simulink model "controller_v13"  (R2020b)
settings: Solver=ode4  StartTime=0.0  StopTime=inf  RelTol=1e-3
undefined symbols (not defined in the file): ctr, DiscIntNeverNeededParam, flt, IO397, mdl, rbt, rsim, som, ukf_P0_flat, ukf_prediction_time, ukf_s0, ukf_sys, ukf_use_prediction
libraries: simulink x31, slrealtimeloglib x5, slrealtimeseriallib x5, speedgoatlib_fpga_analog_io x4, slrealtimetgmanagement x3, speedgoatlib_fpga x2, speedgoatlib_fpga_dio x1, slrealtimeutilitieslib x1
(part 4 of 5)

== matlab function controller_v13/Adaptive Controller/ICRA'23 attitude and thrust MPC controller -> It works/Geometric Attitude Controller ==
  data: time input; cmd_B_torque output; R input; Omega input; Rd input; Omegad input; tau_ext input; ctr parameter; rbt parameter; mdl parameter; att_e output
function [cmd_B_torque, att_e]   = fcn(time, R, Omega, Rd, Omegad, tau_ext, ctr, rbt, mdl)
%#codegen
% r: curr pos
% r_dot: curr vel
% R: current attitude
% Omega: current body rates
% rd : des pos
% rd_d: des vel
% Rd: desired attitude (rotation matrix)
% Omegad: desired angular velocity


% current attitude
R = get_rotation_matrix(R);     % transform vector in rotation matrix
Omega = Omega(:);
Omegad = Omegad(:);

% desired attitude & angvel
Rd = get_rotation_matrix(Rd);
% inertial frame 3-axis



% thrust magnitude control, eq 19
%A = -ctr.lee.pos.kx*ex - ctr.lee.pos.kv*ev - rbt.m*mdl.g*e3; % + P.mass*xd_2dot;
%cmd_B_acc_z = dot(-A, R*e3)/rbt.m;

Rd = get_desired_attitude_x_axis(Rd, R);
%Rd = get_desired_attitude_y_axis(Rd, R);

% inertia matrix
J = diag([ctr.lee.ixx, ctr.lee.iyy, ctr.lee.izz]);

% attitude and angular velocity errors
eR     = (1/2)*vee(Rd.'*R - R.'*Rd);
eOmega = Omega - R.'*Rd*Omegad;
% desired torque
M = -ctr.lee.kR*eR - ctr.lee.kOmega*eOmega + cross(Omega, J*Omega)...
    - J*(hat(Omega)*R.'*Rd*Omegad) ...
    - ctr.torque_obs.factor.*[tau_ext(1); tau_ext(2); 0.0]; % ...
  % - J*(- R.'*Rd*Omegad_1dot);
  % - J*(hat(Omega)*R.'*Rd*Omegad) ...

%att_e = eR'*eR; % squared norm of the error
att_e = eR;
cmd_B_torque = M(:);
end

function vec = vee(ss)
% function vec = vee(skewsymmetric)
%   The vee function maps a skew-symmetric 
%   matrix to a vector

% https://github.com/justinthomas/MATLAB-tools/blob/master/vee.m

if isa(ss,'sym')
    ss = expand(simplify(ss));
end

switch numel(ss)
    
    case 4
        
        if ~isequal(ss(1,2), -ss(2,1))
            disp('The provided matrix is not skew symmetric')
        end
        
        vec = ss(1,2);

    case 9

        if ~isequal(ss(3,2),-ss(2,3)) || ~isequal(ss(1,3),-ss(3,1)) || ~isequal(ss(2,1),-ss(1,2))
            disp('The provided matrix is not skew symmetric.')
            %print(ss)
        end

        vec = [ss(3,2); ss(1,3); ss(2,1)];
end

if isa(ss,'sym')
    vec = simplify(vec);
end

end

function ss = hat(vec)
% function ss = hat(vec)
%   The hat function maps a vector in R^3 (or R^1) to its
%   skew symmetric matrix in R^(3x3) (or R^(2x2))

% https://github.com/justinthomas/MATLAB-tools/blob/master/hat.m

switch length(vec)
    
    case 3
        ss = [...
            0, -vec(3), vec(2);...
            vec(3), 0, -vec(1);...
            -vec(2), vec(1), 0];
        
    case 1
        ss = [...
            0, vec; ...
            -vec, 0];
end

end

function R = get_rotation_matrix(R)
    R11 = R(1);
    R12 = R(2);
    R13 = R(3);
    R21 = R(4);
    R22 = R(5);
    R23 = R(6);
    R31 = R(7);
    R32 = R(8);
    R33 = R(9);
    R1 = [R11; R21; R31];     % unit (column) vector
    R2 = [R12; R22; R32];
    R3 = [R13; R23; R33];
    R = [R1, R2, R3];

end

function Omegad = get_desired_body_velocity()

% time derivatives of body axes -- arXiv:1003.2005v3, Appendix F
A_1dot   = -ctr.lee.pos.kx*ev; %- ctr.lee.pos.kv*ea + ctr.lee.pos.mass*xd_3dot;
b3c_1dot = -A_1dot/norm(A) + (dot(A,A_1dot)/norm(A)^3)*A;
C_1dot   = cross(b3c_1dot, b1d) + cross(b3c, b1d_1dot);
b2c_1dot = C/norm(C) - (dot(C,C_1dot)/norm(C)^3)*C;
% b2c_1dot = -1*b2c_1dot;
b1c_1dot = cross(b2c_1dot, b3c) + cross(b2c, b3c_1dot);

% Extract calculated angular velocities and their time-derivatives
Rd_1dot     = [b1c_1dot b2c_1dot b3c_1dot];
Omegad      = vee(Rd_tmp.'*Rd_1dot);

% Omegad      = [0; 0; 0]; % vee(Rd.'*Rd_1dot);
Omegad_1dot = [0; 0; 0]; % vee(Rd.'*Rd_2dot - hat(Omegad)*hat(Omegad));

end

function Rd = get_desired_attitude_x_axis(Rd, R)

    e3 = [0;0;1];
    % normalized feedback function, eq 23
    b3c = Rd*e3;
    
    % Desired x axis -- current x axis
    b1d = R(:, 1);
    
    % Construct b1c, eq 38
    C = cross(b3c, b1d); % arXiv:1003.2005v3, eq ~97
    b1c = -(1/norm(C))*cross(b3c, C);
    
    b2c = C/norm(C);
    
    % computed attitude, eq 22
    Rd = [b1c b2c b3c];

end


function Rd = get_desired_attitude_y_axis(Rd, R)

    e3 = [0;0;1];
    % normalized feedback function, eq 23
    b3c = Rd*e3;
    
    % Desired y axis -- current x axis
    b2d = R(:, 2);
    
    % Construct b2c, eq 38
    C = cross(b3c, b2d); % arXiv:1003.2005v3, eq ~97
    b2c = -(1/norm(C))*cross(b3c, C);
    
    b1c = C/norm(C);
    
    % computed attitude, eq 22
    Rd = [b1c b2c b3c];

end

== matlab function controller_v13/Adaptive Controller/ICRA'23 attitude and thrust MPC controller -> It works/Geometric Controller ==
  data: time input; r input; Rd output; r_dot input; r_dotdot input; R input; Omega input; rd input; rd_d input; rd_dd input; rd_ddd input; rd_dddd input; int_e input; ctr parameter; rbt parameter; Omegad output; cmd_B_acc_z output; mdl parameter; alt_e output; rd_rtmpc output
function [Rd, Omegad, cmd_B_acc_z, alt_e, rd_rtmpc]   = fcn(time, r, r_dot, r_dotdot, R, Omega, rd,rd_d,rd_dd,rd_ddd,rd_dddd, int_e, ctr, rbt, mdl)
    %#codegen
    % r: curr pos
    % r_dot: curr vel
    % R: current attitude
    % Omega: current body rates
    % rd : des pos
    % rd_d: des vel
    %% Out: 
    % cmd_B_thrust_z is thrust force on z axis in body (B) frame [N]
    
    % Ensure signals have expected shape
    R11 = R(1);
    R12 = R(2);
    R13 = R(3);
    R21 = R(4);
    R22 = R(5);
    R23 = R(6);
    R31 = R(7);
    R32 = R(8);
    R33 = R(9);
    R1 = [R11; R21; R31];     % unit (column) vector
    R2 = [R12; R22; R32];
    R3 = [R13; R23; R33];
    R = [R1, R2, R3];

    r = r(:);           % position
    r_dot = r_dot(:);   % velocity 

    rd = rd(:);         % desired position
    rd_d = rd_d(:);     % desired velocity

    rd_rtmpc = [rd; rd_d];

    
    % From https://github.com/plusk01/se3quad/blob/master/matlab/controller.m
    % calculate errors, eq 17-18
    ex = r - rd;
    ev = r_dot - rd_d;
    %ea = v_1dot - xd_2dot;
    %ej = v_2dot - xd_3dot;
    
    % inertial frame 3-axis
    e3 = [0;0;1];
    
    % thrust magnitude control, eq 19
    A = -ctr.lee.pos.kx*ex - ctr.lee.pos.kv*ev - rbt.m*mdl.g*e3; % + P.mass*xd_2dot;
    cmd_B_acc_z = dot(-A, R*e3)/rbt.m;
    
    % normalized feedback function, eq 23
    b3c = -A/norm(A);

    % Desired x axis -- current x axis
    b1d = R(:, 1);
    % Desired angular velocity of this axis - zero?
    b1d_1dot = [0; 0; 0];
    
    % Construct b1c, eq 38
    C = cross(b3c, b1d); % arXiv:1003.2005v3, eq ~97
    b1c = -(1/norm(C))*cross(b3c, C);
    
    b2c = C/norm(C);
    
    % computed attitude, eq 22
    Rd_tmp = [b1c b2c b3c];

    % time derivatives of body axes -- arXiv:1003.2005v3, Appendix F
    A_1dot   = -ctr.lee.pos.kx*ev; %- ctr.lee.pos.kv*ea + ctr.lee.pos.mass*xd_3dot;
    b3c_1dot = -A_1dot/norm(A) + (dot(A,A_1dot)/norm(A)^3)*A;
    C_1dot   = cross(b3c_1dot, b1d) + cross(b3c, b1d_1dot);
    b2c_1dot = C/norm(C) - (dot(C,C_1dot)/norm(C)^3)*C;
    % b2c_1dot = -1*b2c_1dot;
    b1c_1dot = cross(b2c_1dot, b3c) + cross(b2c, b3c_1dot);
    
    % Extract calculated angular velocities and their time-derivatives
    Rd_1dot     = [b1c_1dot b2c_1dot b3c_1dot];
    Omegad      = vee(Rd_tmp.'*Rd_1dot);

    % Desired angular velocity
    % Omegad = [0.0, 0.0, 0.0]; % TODO

    % Altitude error
    alt_e = r(3) - rd(3); 

    % Generate output. 
    Rd_tmp = Rd_tmp'; % this is needed to respect existing convention that rot. matrices are passed
          % around as vectors, created by concatenating the rows of the
          % matrix (and Rd(:) will created a vector by concatentatig the columns of Rd)
    Rd = Rd_tmp(:);
end

function [B_thrust] = compensate_thrust(cmd_B_acc_z, B_ypr, mass, g)
    B_thrust_z = mass * (cmd_B_acc_z+g)/cos(B_ypr(3))/cos(B_ypr(2));
    B_thrust = [0.0; 0.0; B_thrust_z];
end

function [B_roll, B_pitch] = compensate_attitude(B_thrust, lin_B_roll, lin_B_pitch, mass, g)
    B_acc_z = (B_thrust(3))/mass;
    B_roll = lin_B_roll*(g/B_acc_z);
    B_pitch = lin_B_pitch*(g/B_acc_z);
end

function [R] = get_B_R_yaw_I(yaw)
    R = [cos(yaw), sin(yaw); -sin(yaw), cos(yaw)];
end

function vec = vee(ss)
% function vec = vee(skewsymmetric)
%   The vee function maps a skew-symmetric 
%   matrix to a vector

% https://github.com/justinthomas/MATLAB-tools/blob/master/vee.m

if isa(ss,'sym')
    ss = expand(simplify(ss));
end

switch numel(ss)
    
    case 4
        
        if ~isequal(ss(1,2), -ss(2,1))
            %warning('The provided matrix is not skew symmetric')
        end
        
        vec = ss(1,2);

    case 9

        if ~isequal(ss(3,2),-ss(2,3)) || ~isequal(ss(1,3),-ss(3,1)) || ~isequal(ss(2,1),-ss(1,2))
            %warning('The provided matrix is not skew symmetric.')
            %print(ss)
        end

        vec = [ss(3,2); ss(1,3); ss(2,1)];
end

if isa(ss,'sym')
    vec = simplify(vec);
end

end

== matlab function controller_v13/Adaptive Controller/ICRA'23 attitude and thrust MPC controller -> It works/RTMPC Trajectory Tracking ==
  data: time input; r input; Rd output; r_dot input; r_dotdot input; R input size=9; Omega input; rd input; rd_d input; rd_dd input; rd_ddd input; rd_dddd input; att_cmd input; int_e input; ctr parameter; rbt parameter; Omegad output; cmd_B_acc_z output size=1; mdl parameter; alt_e output; rd_rtmpc output; new_att_cmd output
function [Rd, Omegad, cmd_B_acc_z, alt_e, rd_rtmpc, new_att_cmd]   = fcn(time, r, r_dot, r_dotdot, R, Omega, rd,rd_d,rd_dd,rd_ddd,rd_dddd, att_cmd, int_e, ctr, rbt, mdl)
    %#codegen
    % r: curr pos
    % r_dot: curr vel
    % R: current attitude
    % Omega: current body rates
    % rd : des pos
    % rd_d: des vel
    cmd_B_acc_z = 0;
    %% Out: 
    % cmd_B_thrust_z is thrust force on z axis in body (B) frame [N]
    
    % Ensure signals have expected shape
    R11 = R(1);
    R12 = R(2);
    R13 = R(3);
    R21 = R(4);
    R22 = R(5);
    R23 = R(6);
    R31 = R(7);
    R32 = R(8);
    R33 = R(9);
    R1 = [R11; R21; R31];     % unit (column) vector
    R2 = [R12; R22; R32];
    R3 = [R13; R23; R33];
    R = [R1, R2, R3];

    r = r(:);           % position
    r_dot = r_dot(:);   % velocity 

    rd = rd(:);         % desired position
    rd_d = rd_d(:);     % desired velocity

    new_att_cmd = zeros(2,1);
    Omegad = [0.0; 0.0; 0.0];
    
    % Compute current attitude as euler angles (:( )
    B_ypr = rotm2eul(R);
    B_est_roll = B_ypr(3);
    B_est_pitch = B_ypr(2);
    B_est_yaw = B_ypr(1);

    % Conver attitude in yaw-invariant frame. 
    B_R_yaw_I = get_B_R_yaw_I(B_est_yaw);
    I_rp = B_R_yaw_I'*[B_est_roll; B_est_pitch];

    % Generate reference % (currently only circle is supported)
    x_ref = traj_planner(time, ctr.rtmpc.ref_len, ctr.rtmpc.traj, ctr);

    % Set current state
    x = [r - ctr.rtmpc.r_origin; r_dot; I_rp(1); I_rp(2);];

    if ctr.mode == 0
        % NN RTMPC controller

        % Apply state and reference scaling
        x = [x; att_cmd(1); att_cmd(2)];
        x_scaled = ctr.rtmpc.in_scaling.*x;
        x_ref_scaled = repmat(ctr.rtmpc.in_scaling(1:6), ctr.rtmpc.ref_len, 1).*x_ref;
        
        x_in = [x_scaled; x_ref_scaled];
        x_in = x_in(:); % column vector

        % 10.0 and 12.0 are some scalings applied to the NN to
        % ensure that its input/ouput is in [-1, 1]. 
        % For the rtmpc expert we do not have this care -- but we scale
        % things to ensure that input/outpurs are not too large numbers (e.g., <+-100)
        u_next = 10.0*rtmpcnn(x_in/10.0, ctr.rtmpc.nnparam);

        % Apply rtmpc scaling: 
        u_next = u_next.*ctr.rtmpc.out_scaling;

        % integrated new att cmd
        new_att_cmd = zeros(2,1);
        new_att_cmd(:, 1) = mdl.T*u_next(1:2) + att_cmd;

        % Approach 2: rotate in B after.
        Iy_rp_des_dot = [u_next(1); u_next(2)];
        Iy_rp_des = [new_att_cmd(1); new_att_cmd(2)];
        % compute angular velocity in yaw-aligned frame
        Iy_ypr_des = [0.0; Iy_rp_des(2); Iy_rp_des(1)];
        Iy_ypr_des_dot = [0.0; Iy_rp_des_dot(2); Iy_rp_des_dot(1)];
        Iy_Omegad = get_body_ang_vel(Iy_ypr_des, Iy_ypr_des_dot);
        B_R_yaw_I = get_B_R_yaw_I(B_est_yaw);
        B_Omegad_12 = B_R_yaw_I*Iy_Omegad(1:2);
        Omegad = [B_Omegad_12(1); B_Omegad_12(2); 0.0];
        u_next(1:2) = new_att_cmd;

    elseif ctr.mode == 1
        
        % Set reference 
        %x_ref = [rd; rd_d; 0.0; 0.0]; % no attitude feed-forward at the moment. 
        %mpc.set_reference_trajectory(x_ref);
    
        % Compute new linearized commands
        x = [r; r_dot; I_rp(1); I_rp(2)];

        x_scaled = x.*ctr.lqrv2.in_scaling;
        x_ref_scaled = [x_ref(1:6); 0.0; 0.0;].*ctr.lqrv2.in_scaling;
        u_next = -ctr.lqrv2.K*(x_scaled - x_ref_scaled);
        u_next = u_next.*ctr.lqrv2.out_scaling;
        Omegad = zeros(3, 1);

    elseif ctr.mode == 2
        x = [x; att_cmd(1); att_cmd(2)];
        ctr.lqr.in_scaling = [10; 10; 10; 10; 10; 10; 1; 1; 1; 1];
        x_scaled = x.*ctr.lqr.in_scaling;
        x_ref_scaled = [x_ref(1:6); 0.0; 0.0; 0.0; 0.0;].*ctr.lqr.in_scaling;
        u_next = -ctr.lqr.K*(x_scaled - x_ref_scaled);
        u_next = u_next.*ctr.lqr.out_scaling;

        % integrated new att cmd
        new_att_cmd = zeros(2,1);
        new_att_cmd(:, 1) = mdl.T*u_next(1:2,1) + att_cmd;

        % Approach 1: rotate in B first.
%         I_rp_des_dot = [u_next(1); u_next(2)];
%         B_R_yaw_I = get_B_R_yaw_I(B_est_yaw);
%         B_rp_des_dot = B_R_yaw_I*I_rp_des_dot;
%         B_ypr_des = [B_ypr(1); new_att_cmd(2); new_att_cmd(1)];
%         B_ypr_des_dot = [0.0; B_rp_des_dot(2); B_rp_des_dot(1)];
%         %Omegad = [B_ypr_des_dot(3); B_ypr_des_dot(2); B_ypr_des_dot(1)];
%         Omegad = get_body_ang_vel(B_ypr_des, B_ypr_des_dot);
%         u_next(1:2) = new_att_cmd;

%         % Approach 2: rotate in B after.
        Iy_rp_des_dot = [u_next(1); u_next(2)];
        Iy_rp_des = [new_att_cmd(1); new_att_cmd(2)];
        % compute angular velocity in yaw-aligned frame
        Iy_ypr_des = [0.0; Iy_rp_des(2); Iy_rp_des(1)];
        Iy_ypr_des_dot = [0.0; Iy_rp_des_dot(2); Iy_rp_des_dot(1)];
        Iy_Omegad = get_body_ang_vel(Iy_ypr_des, Iy_ypr_des_dot);
        B_R_yaw_I = get_B_R_yaw_I(B_est_yaw);
        B_Omegad_12 = B_R_yaw_I*Iy_Omegad(1:2);
        Omegad = [B_Omegad_12(1); B_Omegad_12(2); 0.0];
        u_next(1:2) = new_att_cmd;

    else
        disp("ctr.mode not recognized. ")
        u_next= zeros(3, 1);
    end

    rd_rtmpc = x_ref(1:6);
    rd_rtmpc(1:3) = rd_rtmpc(1:3) + ctr.rtmpc.r_origin;
    
    delta_cmd_I_roll =  u_next(1);
    delta_cmd_I_pitch = u_next(2);
    delta_cmd_I_acc_z = u_next(3);
    
    % Compensate thrust
    cmd_B_thrust = compensate_thrust(delta_cmd_I_acc_z, B_ypr, rbt.m, mdl.g);
    cmd_B_thrust_z = cmd_B_thrust(3);
    cmd_B_acc_z = cmd_B_thrust_z/rbt.m;
   
    % apply saturation
    cmd_B_acc_z = max(min(cmd_B_acc_z, mdl.g+2.0), mdl.g-1.0);
    
    % De-rotate attitude commands in body frame
    cmd_I_rp = [delta_cmd_I_roll; delta_cmd_I_pitch];
    B_R_yaw_I = get_B_R_yaw_I(B_est_yaw);
    cmd_B_rp = B_R_yaw_I*cmd_I_rp;

    % Compensate attitude
    if ctr.rtmpc.compensate_attitude
        [cmd_B_roll, cmd_B_pitch] = compensate_attitude(cmd_B_thrust, cmd_B_rp(1), cmd_B_rp(2), rbt.m, mdl.g);
    else
        cmd_B_roll = cmd_B_rp(1);
        cmd_B_pitch = cmd_B_rp(2);
    end
    cmd_B_roll = max(min(cmd_B_roll, ctr.rtmpc.lim.att), -ctr.rtmpc.lim.att);
    cmd_B_pitch = max(min(cmd_B_pitch, ctr.rtmpc.lim.att), -ctr.rtmpc.lim.att);
    cmd_B_yaw = B_est_yaw;

    % Desired angular velocity
    % Omegad = [0.0, 0.0, 0.0]; % TODO
   

    % Altitude error
    alt_e = r(3) - rd(3); 

    freq = 0.25*time;
    %cmd_B_roll = pi/6*square(time*freq);
    %cmd_B_pitch = pi/6*square(time*freq - pi/2);

    %cmd_B_roll = 0.0;
    %cmd_B_pitch = 0.0;
    %cmd_B_yaw = pi/2;
    
    % Desired attitude from RTMPC as rotation matrix
    Rd_tmp = eul2rotm([cmd_B_yaw, cmd_B_pitch, cmd_B_roll]); % intrinsic, zyx


    % Eq 15 of Lee2010: treat I_T from mpc as (-kxex -kvev - mge3 + mxdd):
    %e3 = [0; 0; 1];
    %cmd_B_acc_z = (Rd_tmp*[0; 0; cmd_B_acc_z])'*R*e3;

%     %%% TODO: Andrea: remove
%     % Try flip
%     speedf = 5.0;
%     if (time > 1.0) && (time < (1.0 + 1.0/speedf))
%         Rd_tmp = axang2rotm([-1, 0, 0, speedf*2.0*pi*(1.0 - time)]);
%         Omegad = [speedf*2.0*pi, 0.0, 0.0];
%     end
%     %%% 

    % Generate output. 
    Rd_tmp = Rd_tmp'; % this is needed to respect existing convention that rot. matrices are passed
          % around as vectors, created by concatenating the rows of the
          % matrix (and Rd(:) will created a vector by concatentatig the columns of Rd)
    Rd = Rd_tmp(:);
end

function [B_thrust] = compensate_thrust(cmd_B_acc_z, B_ypr, mass, g)
    B_thrust_z = mass * (cmd_B_acc_z+g)/cos(B_ypr(3))/cos(B_ypr(2));
    B_thrust = [0.0; 0.0; B_thrust_z];
end

function [B_roll, B_pitch] = compensate_attitude(B_thrust, lin_B_roll, lin_B_pitch, mass, g)
    B_acc_z = (B_thrust(3))/mass;
    B_roll = lin_B_roll*(g/B_acc_z);
    B_pitch = lin_B_pitch*(g/B_acc_z);
end

function [R] = get_B_R_yaw_I(yaw)
    R = [cos(yaw), sin(yaw); -sin(yaw), cos(yaw)];
end

function [B_omega] = get_body_ang_vel(B_ypr, B_ypr_dot)
% https://www.astro.rug.nl/software/kapteyn-beta/_downloads/attitude.pdf
sy = sin(B_ypr(1));
cy = cos(B_ypr(1));
sp = sin(B_ypr(2));
cp = cos(B_ypr(2));
E_zyx = [[0; 0; 1], [-sy; cy; 0.0], [cy*cp; sy*cp; -sp]];
B_omega = E_zyx*B_ypr_dot;

end

== matlab function controller_v13/Adaptive Controller/ICRA'23 attitude and thrust MPC controller -> It works/Rotm2rpy ==
  data: R input; rpy output size=3
function rpy  = fcn(R)
    R = get_rotation_matrix(R);
    ypr = rotm2eul(R); 
    rpy = squeeze([ypr(3); ypr(2); ypr(1)]);

end

function R = get_rotation_matrix(R)
    R11 = R(1);
    R12 = R(2);
    R13 = R(3);
    R21 = R(4);
    R22 = R(5);
    R23 = R(6);
    R31 = R(7);
    R32 = R(8);
    R33 = R(9);
    R1 = [R11; R21; R31];     % unit (column) vector
    R2 = [R12; R22; R32];
    R3 = [R13; R23; R33];
    R = [R1, R2, R3];
end

== matlab function controller_v13/Adaptive Controller/ICRA'23 attitude and thrust MPC controller -> It works/Rotm2rpy1 ==
  data: R input; rpy output size=3
function rpy   = fcn(R)
    R = get_rotation_matrix(R);
    ypr = rotm2eul(R); 
    rpy = [ypr(3); ypr(2); ypr(1)];
end

function R = get_rotation_matrix(R)
    R11 = R(1);
    R12 = R(2);
    R13 = R(3);
    R21 = R(4);
    R22 = R(5);
    R23 = R(6);
    R31 = R(7);
    R32 = R(8);
    R33 = R(9);
    R1 = [R11; R21; R31];     % unit (column) vector
    R2 = [R12; R22; R32];
    R3 = [R13; R23; R33];
    R = [R1, R2, R3];
end

== matlab function controller_v13/Adaptive Controller/ICRA'23 attitude and thrust MPC controller -> It works/MATLAB Function ==
  data: Tx input; Tx_out output; Ty input; time input; Ty_out output; mdl parameter; ctr parameter
function [Tx_out, Ty_out] = fcn(Tx, Ty, time, mdl, ctr)

if time > mdl.i_delay && ctr.en
    Tx_out = Tx;
    Ty_out = Ty;
else
    Tx_out = 0;
    Ty_out = 0;
end

end

== matlab function controller_v13/Adaptive Controller/observer/Linear Observer (ICRA'23)/lateral KF observer/Translational Dynamics & Kinamatics Lin Obs ==
  data: R input; pos_hat output; f_cmd input; meas_pos input; pos_hat input; vel_hat input; vel_hat output; ctr parameter; rbt parameter; acc_hat output; mdl parameter; id_in input; id_out output
function [pos_hat, vel_hat, acc_hat, id_out] = fcn(R, f_cmd, meas_pos, pos_hat, vel_hat, ctr, rbt, mdl, id_in)


pos_hat = pos_hat(:);
vel_hat = vel_hat(:);
meas_pos = meas_pos(:);
R11 = R(1);
R12 = R(2);
R13 = R(3);
R21 = R(4);
R22 = R(5);
R23 = R(6);
R31 = R(7);
R32 = R(8);
R33 = R(9);
R1 = [R11; R21; R31];     % unit (column) vector
R2 = [R12; R22; R32];
R3 = [R13; R23; R33];
R = [R1, R2, R3];



if ctr.en
    u = (R*[0; 0; f_cmd] - [0; 0; rbt.m*mdl.g])/rbt.m;
else
    u = [0; 0; 0]; 
end

u = (R*[0; 0; f_cmd] - [0; 0; rbt.m*mdl.g])/rbt.m;
x_hat_curr = [pos_hat(:); vel_hat(:)];
y = meas_pos; 
x_hat_pred = ctr.pos_vel_est.A*x_hat_curr + ctr.pos_vel_est.B(:, 1:3)*u; 
x_hat_next = (x_hat_pred + ctr.pos_vel_est.L*(y - ctr.pos_vel_est.C*x_hat_pred));

pos_hat = x_hat_next(1:3);
vel_hat = x_hat_next(4:6);
acc_hat = u;

pos_hat = pos_hat(:);
vel_hat = vel_hat(:);
acc_hat = acc_hat(:);

if id_in < 4
    pos_hat = meas_pos;
end

id_out = id_in + 1;

end

== matlab function controller_v13/Adaptive Controller/observer/UKF/UKF1/R_flat to quat ==
  data: R_flat input; q output
function q = fcn(R_flat)
% convertion from rotation matrix to quaternion
q = rotm2quat(UKF.unflatten_matrix(R_flat))';
end

== matlab function controller_v13/Adaptive Controller/observer/UKF/UKF1/UKF_inner/UKF update then predict ==
  data: s_out output; z_raw input; z_raw_prev input; f_cmd input; tau_cmd_x input; tau_cmd_y input; s_in input; P_in_flat input; is_init_in input; s_prediction_time input; sys parameter; P_out_flat output; is_init_out output; s_out_pre output; s_prediction_out output; md output
function [s_out, P_out_flat, is_init_out, s_out_pre, s_prediction_out, md] = fcn(z_raw, z_raw_prev, f_cmd, tau_cmd_x, tau_cmd_y, s_in, P_in_flat, is_init_in, s_prediction_time, sys)
    [s_out, P_out_flat, is_init_out, s_out_pre, s_prediction_out, md] = UKF.inner_helper(z_raw, z_raw_prev, f_cmd, tau_cmd_x, tau_cmd_y, s_in, P_in_flat, is_init_in, s_prediction_time, sys);
end

== matlab function controller_v13/Adaptive Controller/observer/UKF/UKF/UKF_inner/UKF update then predict ==
  data: s_out output; z_raw input; z_raw_prev input; f_cmd input; tau_cmd_x input; tau_cmd_y input; s_in input; P_in_flat input; is_init_in input; sys parameter; P_out_flat output; is_init_out output
function [s_out, P_out_flat, is_init_out] = fcn(z_raw, z_raw_prev, f_cmd, tau_cmd_x, tau_cmd_y, s_in, P_in_flat, is_init_in, sys)
    [s_out, P_out_flat, is_init_out] = UKF.inner_helper(z_raw, z_raw_prev, f_cmd, tau_cmd_x, tau_cmd_y, s_in, P_in_flat, is_init_in, sys);
end

== matlab function controller_v13/Adaptive Controller/observer/UKF/UKF/euler to quat ==
  data: euler_angles input; q output
function q = fcn(euler_angles)
% convertion from euler to R block

eu_x = euler_angles(1);
eu_y = euler_angles(2);
eu_z = euler_angles(3);

R = [cos(eu_y)*cos(eu_z); -cos(eu_y)*sin(eu_z); sin(eu_y); ...
    cos(eu_x)*sin(eu_z)+sin(eu_x)*sin(eu_y)*cos(eu_z); cos(eu_x)*cos(eu_z)-sin(eu_x)*sin(eu_y)*sin(eu_z); -sin(eu_x)*cos(eu_y); ...
    sin(eu_x)*sin(eu_z)-cos(eu_x)*sin(eu_y)*cos(eu_z); sin(eu_x)*cos(eu_z)+cos(eu_x)*sin(eu_y)*sin(eu_z); cos(eu_x)*cos(eu_y)];
% R is 1x9

R_unflattened = UKF.unflatten_matrix(R);
q = rotm2quat(R_unflattened)';
      


end

== matlab function controller_v13/Adaptive Controller/observer/UKF/UKF/quaternion to rotation matrix ==
  data: q input; R_flat output
function R_flat = fcn(q)
    % Assume q = [q_s; q_x, q_y, q_z];
    R = quat2rotm(q');
    R_flat = UKF.flatten_matrix(R);
end

== matlab function controller_v13/Adaptive Controller/observer/UKF/UKF1/pack measurement vector ==
  data: r input; z_raw output; q input
function z_raw = fcn(r, q)
    z_raw = vertcat(r, q, zeros(6,1));
end

== matlab function controller_v13/Adaptive Controller/observer/UKF/UKF1/quaternion to rotation matrix ==
  data: q input; R_flat output
function R_flat = fcn(q)
    % Assume q = [q_s; q_x, q_y, q_z];
    R = quat2rotm(q');
    R_flat = UKF.flatten_matrix(R);
end

== matlab function controller_v13/Adaptive Controller/attitude and thrust MPC controller2/MATLAB Function1 ==
  data: u input; y output
function y = fcn(u)

y = u;

== matlab function controller_v13/Adaptive Controller/attitude and thrust MPC controller2/NN RTMPC/MATLAB Function ==
  data: time input; x_in output; r input; r_dot input; r_dotdot input; R input; Omega input; rd input; rd_d input; rd_dd input; rd_ddd input; rd_dddd input; int_e input; mdl parameter; rbt parameter; ctr parameter
function x_in    = fcn(time, r, r_dot, r_dotdot, R, Omega, rd,rd_d,rd_dd,rd_ddd,rd_dddd, int_e, mdl, rbt, ctr)
    %#codegen
    % r: curr pos
    % r_dot: curr vel
    % R: current attitude
    % Omega: current body rates
    % rd : des pos
    % rd_d: des vel
    %% Out: 
    % cmd_B_thrust_z is thrust force on z axis in body (B) frame [N]
    
    % Ensure signals have expected shape
    R11 = R(1);
    R12 = R(2);
    R13 = R(3);
    R21 = R(4);
    R22 = R(5);
    R23 = R(6);
    R31 = R(7);
    R32 = R(8);
    R33 = R(9);
    R1 = [R11; R21; R31];     % unit (column) vector
    R2 = [R12; R22; R32];
    R3 = [R13; R23; R33];
    R = [R1, R2, R3];

    r = r(:);           % position
    r_dot = r_dot(:);   % velocity 

    rd = rd(:);         % desired position
    rd_d = rd_d(:);     % desired velocity
    
    % Compute current attitude as euler angles (:( )
    B_ypr = rotm2eul(R);
    B_est_roll = B_ypr(3);
    B_est_pitch = B_ypr(2);
    B_est_yaw = B_ypr(1);

    % Conver attitude in yaw-invariant frame. 
    B_R_yaw_I = get_B_R_yaw_I(B_est_yaw);
    I_rp = B_R_yaw_I'*[B_est_roll; B_est_pitch];

    % Set reference 
    x_ref_t0 = [rd; rd_d;]; % no attitude feed-forward at the moment. 
    x_ref = repmat(x_ref_t0, 20, 1);
    %mpc.set_reference_trajectory(x_ref);
    
    % Set current state
    x = [r; r_dot; I_rp(1); I_rp(2)];

    x_in = [x; x_ref];
    x_in = x_in(:); % column vector
    
end

function [R] = get_B_R_yaw_I(yaw)
    R = [cos(yaw), sin(yaw); -sin(yaw), cos(yaw)];
end

== matlab function controller_v13/Adaptive Controller/attitude and thrust MPC controller2/NN RTMPC/MATLAB Function1 ==
  data: u_nn input; Rd output; Omegad output; cmd_B_acc_z output; alt_e output; R input; rbt input; mdl input
function [Rd, Omegad, cmd_B_acc_z, alt_e] = fcn(u_nn, R, rbt, mdl)
    %#codegen
    % r: curr pos
    % r_dot: curr vel
    % R: current attitude
    % Omega: current body rates
    % rd : des pos
    % rd_d: des vel
    %% Out: 
    % cmd_B_thrust_z is thrust force on z axis in body (B) frame [N]
    
    % Ensure signals have expected shape
    R11 = R(1);
    R12 = R(2);
    R13 = R(3);
    R21 = R(4);
    R22 = R(5);
    R23 = R(6);
    R31 = R(7);
    R32 = R(8);
    R33 = R(9);
    R1 = [R11; R21; R31];     % unit (column) vector
    R2 = [R12; R22; R32];
    R3 = [R13; R23; R33];
    R = [R1, R2, R3];

    u_nn = u_nn(:);
    
    % Compute current attitude as euler angles (:( )
    B_ypr = rotm2eul(R);
    B_est_roll = B_ypr(3);
    B_est_pitch = B_ypr(2);
    B_est_yaw = B_ypr(1);

    % Conver attitude in yaw-invariant frame. 
    B_R_yaw_I = get_B_R_yaw_I(B_est_yaw);
    I_rp = B_R_yaw_I'*[B_est_roll; B_est_pitch];
    
    delta_cmd_I_roll =  u_nn(1);
    delta_cmd_I_pitch = u_nn(2);
    delta_cmd_I_acc_z = u_nn(3);
    
    % Compensate thrust
    cmd_B_thrust = compensate_thrust(delta_cmd_I_acc_z, B_ypr, rbt.m, mdl.g);
    cmd_B_thrust_z = cmd_B_thrust(3);
    cmd_B_acc_z = cmd_B_thrust_z/rbt.m;
    
    % De-rotate attitude commands in body frame
    cmd_I_rp = [delta_cmd_I_roll; delta_cmd_I_pitch];
    B_R_yaw_I = get_B_R_yaw_I(B_est_yaw);
    cmd_B_rp = B_R_yaw_I*cmd_I_rp;
    
    % Compensate attitude
    [cmd_B_roll, cmd_B_pitch] = compensate_attitude(cmd_B_thrust, cmd_B_rp(1), cmd_B_rp(2), rbt.m, mdl.g);

    % Desired angular velocity
    Omegad = [0.0, 0.0, 0.0]; % TODO

    cmd_B_roll  = cmd_B_rp(1); 
    cmd_B_pitch = cmd_B_rp(2);
    cmd_B_yaw = 0.0*B_est_yaw;

    % Altitude error
    alt_e = r(3) - rd(3); 
    
    % Desired attitude as rotation matrix
    Rd_tmp = eul2rotm([cmd_B_yaw, cmd_B_pitch, cmd_B_roll]);

    
%     %%% TODO: Andrea: remove
%     % Try flip
%     speedf = 5.0;
%     if (time > 1.0) && (time < (1.0 + 1.0/speedf))
%         Rd_tmp = axang2rotm([-1, 0, 0, speedf*2.0*pi*(1.0 - time)]);
%         Omegad = [speedf*2.0*pi, 0.0, 0.0];
%     end
%     %%% 

    % Generate output. 
    Rd_tmp = Rd_tmp'; % this is needed to respect existing convention that rot. matrices are passed
          % around as vectors, created by concatenating the rows of the
          % matrix (and Rd(:) will created a vector by concatentatig the columns of Rd)
    Rd = Rd_tmp(:);
end

function [B_thrust] = compensate_thrust(cmd_B_acc_z, B_ypr, mass, g)
    B_thrust_z = mass * (cmd_B_acc_z+g)/cos(B_ypr(3))/cos(B_ypr(2));
    B_thrust = [0.0; 0.0; B_thrust_z];
end

function [B_roll, B_pitch] = compensate_attitude(B_thrust, lin_B_roll, lin_B_pitch, mass, g)
    B_acc_z = (B_thrust(3))/mass;
    B_roll = lin_B_roll*(g/B_acc_z);
    B_pitch = lin_B_pitch*(g/B_acc_z);
end

function [R] = get_B_R_yaw_I(yaw)
    R = [cos(yaw), sin(yaw); -sin(yaw), cos(yaw)];
end

== matlab function controller_v13/Adaptive Controller/attitude and thrust MPC controller2/NN RTMPC/MATLAB Function2 ==
  data: x input; y output; nnparam parameter
function y = fcn(x, nnparam)
    y = rtmpcnn(x, nnparam)
end

== matlab function controller_v13/Adaptive Controller/observer/Linear Observer (ICRA'23)/Rotaion/Rotation Matrix1 ==
  data: R input; Rdot input; w output
function w  = fcn(R,Rdot)
%#codegen
w = zeros(3,1);
w(1) = R(3)*Rdot(2) + R(6)*Rdot(5) + R(9)*Rdot(8);
w(2) = R(1)*Rdot(3) + R(4)*Rdot(6) + R(7)*Rdot(9);
w(3) = R(2)*Rdot(1) + R(5)*Rdot(4) + R(8)*Rdot(7);

== matlab function controller_v13/Adaptive Controller/attitude and thrust MPC controller2/RTMPC Trajectory Tracking ==
  data: time input; r input; Rd output; r_dot input; r_dotdot input; R input; Omega input; rd input; rd_d input; rd_dd input; rd_ddd input; rd_dddd input; int_e input; ctr parameter; rbt parameter; Omegad output; cmd_B_acc_z output; mdl parameter; alt_e output; rd_rtmpc output
function [Rd, Omegad, cmd_B_acc_z, alt_e, rd_rtmpc]   = fcn(time, r, r_dot, r_dotdot, R, Omega, rd,rd_d,rd_dd,rd_ddd,rd_dddd, int_e, ctr, rbt, mdl)
    %#codegen
    % r: curr pos
    % r_dot: curr vel
    % R: current attitude
    % Omega: current body rates
    % rd : des pos
    % rd_d: des vel
    %% Out: 
    % cmd_B_thrust_z is thrust force on z axis in body (B) frame [N]
    
    % Ensure signals have expected shape
    R11 = R(1);
    R12 = R(2);
    R13 = R(3);
    R21 = R(4);
    R22 = R(5);
    R23 = R(6);
    R31 = R(7);
    R32 = R(8);
    R33 = R(9);
    R1 = [R11; R21; R31];     % unit (column) vector
    R2 = [R12; R22; R32];
    R3 = [R13; R23; R33];
    R = [R1, R2, R3];

    r = r(:);           % position
    r_dot = r_dot(:);   % velocity 

    rd = rd(:);         % desired position
    rd_d = rd_d(:);     % desired velocity
    
    % Compute current attitude as euler angles (:( )
    B_ypr = rotm2eul(R);
    B_est_roll = B_ypr(3);
    B_est_pitch = B_ypr(2);
    B_est_yaw = B_ypr(1);

    % Conver attitude in yaw-invariant frame. 
    B_R_yaw_I = get_B_R_yaw_I(B_est_yaw);
    I_rp = B_R_yaw_I'*[B_est_roll; B_est_pitch];

    % Set reference 
    x_ref = [rd; rd_d; 0.0; 0.0]; % no attitude feed-forward at the moment. 
    %mpc.set_reference_trajectory(x_ref);
    
    % Compute new linearized commands
    x = [r; r_dot; I_rp(1); I_rp(2)];

    % Generate reference % (currently only circle is supported)
    x_ref = traj_planner(time, ctr.rtmpc.ref_len, ctr.rtmpc.traj);

    % Set current state
    x = [r - ctr.rtmpc.r_origin; r_dot; I_rp(1); I_rp(2)];

    if ctr.rtmpc.en
        % Set reference - constant
        % x_ref_t0 = [rd - ctr.rtmpc.r_origin; rd_d;]; % no attitude feed-forward at the moment. 
        % x_ref = repmat(x_ref_t0, 20, 1);

        % Set reference - circle
        % Apply state and reference scaling
        x_scaled = ctr.rtmpc.in_scaling.*x;
        x_ref_scaled = repmat(ctr.rtmpc.in_scaling(1:6), ctr.rtmpc.ref_len, 1).*x_ref;
        
        x_in = [x_scaled; x_ref_scaled];
        x_in = x_in(:); % column vector

        % 10.0 and 12.0 are some scalings applied to the NN to
        % ensure that its input/ouput is in [-1, 1]. 
        % For the rtmpc expert we do not have this care -- but we scale
        % things to ensure that input/outpurs are not too large numbers (e.g., <+-100)
        u_next = 12.0*rtmpcnn(x_in/10.0, ctr.rtmpc.nnparam);

        % Apply rtmpc scaling: 
        u_next = u_next.*ctr.rtmpc.out_scaling;

    else
        x_scaled = x.*ctr.lqr.in_scaling;
        x_ref_scaled = [x_ref(1:6); 0.0; 0.0].*ctr.lqr.in_scaling;
        u_next = -ctr.lqr.K*(x_scaled - x_ref_scaled);
        u_next = u_next.*ctr.lqr.out_scaling;
    end

    rd_rtmpc = x_ref(1:6);
    
    delta_cmd_I_roll =  u_next(1);
    delta_cmd_I_pitch = u_next(2);
    delta_cmd_I_acc_z = u_next(3);
    
    % Compensate thrust
    cmd_B_thrust = compensate_thrust(delta_cmd_I_acc_z, B_ypr, rbt.m, mdl.g);
    cmd_B_thrust_z = cmd_B_thrust(3);
    cmd_B_acc_z = cmd_B_thrust_z/rbt.m;
   
    % apply saturation
    cmd_B_acc_z = max(min(cmd_B_acc_z, mdl.g*1.4), mdl.g*0.7);
    
    % De-rotate attitude commands in body frame
    cmd_I_rp = [delta_cmd_I_roll; delta_cmd_I_pitch];
    B_R_yaw_I = get_B_R_yaw_I(B_est_yaw);
    cmd_B_rp = B_R_yaw_I*cmd_I_rp;
    
    % Compensate attitude
    [cmd_B_roll, cmd_B_pitch] = compensate_attitude(cmd_B_thrust, cmd_B_rp(1), cmd_B_rp(2), rbt.m, mdl.g);
    cmd_B_roll = max(min(cmd_B_roll, ctr.rtmpc.lim.att), -ctr.rtmpc.lim.att);
    cmd_B_pitch = max(min(cmd_B_pitch, ctr.rtmpc.lim.att), -ctr.rtmpc.lim.att);
    cmd_B_yaw = B_est_yaw;

    % Desired angular velocity
    Omegad = [0.0, 0.0, 0.0]; % TODO

    % Altitude error
    alt_e = r(3) - rd(3); 
    
    % Desired attitude as rotation matrix
    Rd_tmp = eul2rotm([cmd_B_yaw, cmd_B_pitch, cmd_B_roll]);

    
%     %%% TODO: Andrea: remove
%     % Try flip
%     speedf = 5.0;
%     if (time > 1.0) && (time < (1.0 + 1.0/speedf))
%         Rd_tmp = axang2rotm([-1, 0, 0, speedf*2.0*pi*(1.0 - time)]);
%         Omegad = [speedf*2.0*pi, 0.0, 0.0];
%     end
%     %%% 

    % Generate output. 
    Rd_tmp = Rd_tmp'; % this is needed to respect existing convention that rot. matrices are passed
          % around as vectors, created by concatenating the rows of the
          % matrix (and Rd(:) will created a vector by concatentatig the columns of Rd)
    Rd = Rd_tmp(:);
end

function [B_thrust] = compensate_thrust(cmd_B_acc_z, B_ypr, mass, g)
    B_thrust_z = mass * (cmd_B_acc_z+g)/cos(B_ypr(3))/cos(B_ypr(2));
    B_thrust = [0.0; 0.0; B_thrust_z];
end

function [B_roll, B_pitch] = compensate_attitude(B_thrust, lin_B_roll, lin_B_pitch, mass, g)
    B_acc_z = (B_thrust(3))/mass;
    B_roll = lin_B_roll*(g/B_acc_z);
    B_pitch = lin_B_pitch*(g/B_acc_z);
end

function [R] = get_B_R_yaw_I(yaw)
    R = [cos(yaw), sin(yaw); -sin(yaw), cos(yaw)];
end

== matlab function controller_v13/Adaptive Controller/attitude and thrust MPC controller2/Rotm2rpy ==
  data: R input; rpy output size=3
function rpy  = fcn(R)
    R = get_rotation_matrix(R);
    ypr = rotm2eul(R); 
    rpy = squeeze([ypr(3); ypr(2); ypr(1)]);

end

function R = get_rotation_matrix(R)
    R11 = R(1);
    R12 = R(2);
    R13 = R(3);
    R21 = R(4);
    R22 = R(5);
    R23 = R(6);
    R31 = R(7);
    R32 = R(8);
    R33 = R(9);
    R1 = [R11; R21; R31];     % unit (column) vector
    R2 = [R12; R22; R32];
    R3 = [R13; R23; R33];
    R = [R1, R2, R3];
end

== matlab function controller_v13/Adaptive Controller/attitude and thrust MPC controller2/Rotm2rpy1 ==
  data: R input; rpy output size=3
function rpy   = fcn(R)
    R = get_rotation_matrix(R);
    ypr = rotm2eul(R); 
    rpy = [ypr(3); ypr(2); ypr(1)];
end

function R = get_rotation_matrix(R)
    R11 = R(1);
    R12 = R(2);
    R13 = R(3);
    R21 = R(4);
    R22 = R(5);
    R23 = R(6);
    R31 = R(7);
    R32 = R(8);
    R33 = R(9);
    R1 = [R11; R21; R31];     % unit (column) vector
    R2 = [R12; R22; R32];
    R3 = [R13; R23; R33];
    R = [R1, R2, R3];
end

== matlab function controller_v13/Adaptive Controller/observer/UKF/UKF1/UKF_inner/bee units to SI ==
  data: s_bee input; s_si output
function s_si  = fcn(s_bee)
    s_si = UKF.s_bee_to_s_si(s_bee);
end

== matlab function controller_v13/Adaptive Controller/observer/UKF/UKF/pack measurement vector ==
  data: r input; z_raw output; q input; r_dot input; omega input
function z_raw = fcn(r, q, r_dot, omega)
    z_raw = vertcat(r, q, r_dot, omega);
end

== matlab function controller_v13/Adaptive Controller/observer/UKF/UKF/unpack state vector ==
  data: s input; r output; q output; r_dot output; omega output
function [r, q, r_dot, omega] = fcn(s)
    [r, q, r_dot, omega] = UKF.partial_unpack_s(s);
end

== matlab function controller_v13/Adaptive Controller/observer/UKF/UKF1/UKF_inner/bee cov to SI cov ==
  data: P_flat_bee input; P_flat_si output
function P_flat_si  = fcn(P_flat_bee)
    P_flat_si = UKF.flatten_matrix(diag(UKF.var_bee_to_var_si(diag(UKF.unflatten_matrix(P_flat_bee)))));
end

== matlab function controller_v13/Adaptive Controller/observer/UKF/UKF1/UKF_inner/bee units to SI1 ==
  data: s_bee input; s_si output
function s_si  = fcn(s_bee)
    s_si = UKF.s_bee_to_s_si(s_bee);
end

== matlab function controller_v13/Adaptive Controller/attitude and thrust controller1/Attitude Controleller ==
  data: r input; torque_x output size=1; r_dot input; r_dotdot input; R input; Omega input; rd input; rd_d input; rd_dd input; rd_ddd input; rd_dddd input; int_e input; ctr parameter; rbt parameter; torque_y output size=1; torque_z output size=1; att_e output size=3; mdl parameter
 function [torque_x, torque_y, torque_z, att_e] = fcn(r, r_dot, r_dotdot, R, Omega, rd,rd_d,rd_dd,rd_ddd,rd_dddd, int_e, ctr, rbt, mdl)
%#codegen

%% init
R11 = R(1);
R12 = R(2);
R13 = R(3);
R21 = R(4);
R22 = R(5);
R23 = R(6);
R31 = R(7);
R32 = R(8);
R33 = R(9);
R1 = [R11; R21; R31];     % unit (column) vector
R2 = [R12; R22; R32];
R3 = [R13; R23; R33];
wx = Omega(1);
wy = Omega(2);
wz = Omega(3);

Dr = r-rd;
Dr_dot = r_dot-rd_d;

torque_x = -dot(R2,rd_dddd) - ...
    ctr.gain.at3*( mdl.g*wx+dot(R2,rd_ddd) ) - ...
    ctr.gain.at2*( dot(R2,mdl.g*[0;0;1]+rd_dd) ) + ...
    ctr.gain.at1*( dot(R2,Dr_dot) ) + ...
    ctr.gain.at0*( dot(R2,Dr) ) + ...
    ctr.gain.ati*( int_e(1) );
torque_x = torque_x*rbt.ixx/mdl.g;

torque_y = dot(R1,rd_dddd) - ...
    ctr.gain.at3*( mdl.g*wy-dot(R1,rd_ddd) ) - ...
    ctr.gain.at2*( dot(R1,-mdl.g*[0;0;1]-rd_dd) ) - ...
    ctr.gain.at1*( dot(R1,Dr_dot) ) - ...
    ctr.gain.at0*( dot(R1,Dr) ) + ...
    ctr.gain.ati*( int_e(2) );

torque_y = torque_y*rbt.iyy/mdl.g;

torque_z = 0;           % no yaw control

att_e = -[-dot(R2,Dr);dot(R1,Dr);0];

== matlab function controller_v13/Adaptive Controller/observer/UKF/UKF1/unpack state ==
  data: s input; r output; q output; r_dot output; omega output; F_ext output; tau_ext output
function [r, q, r_dot, omega, F_ext, tau_ext] = fcn(s)
    [r, q, r_dot, omega, F_ext, tau_ext] = UKF.unpack_s(s);
end

== matlab function controller_v13/Adaptive Controller/observer/UKF/UKF2/UKF_inner/UKF update then predict ==
  data: s_out output; z_raw input; z_raw_prev input; f_cmd input; tau_cmd_x input; tau_cmd_y input; s_in input; P_in_flat input; is_init_in input; sys parameter; P_out_flat output; is_init_out output
function [s_out, P_out_flat, is_init_out] = fcn(z_raw, z_raw_prev, f_cmd, tau_cmd_x, tau_cmd_y, s_in, P_in_flat, is_init_in, sys)
    [s_out, P_out_flat, is_init_out] = UKF.inner_helper(z_raw, z_raw_prev, f_cmd, tau_cmd_x, tau_cmd_y, s_in, P_in_flat, is_init_in, sys);
end

== matlab function controller_v13/Adaptive Controller/observer/UKF/UKF2/euler to quat ==
  data: euler_angles input; q output
function q = fcn(euler_angles)
% convertion from euler to R block

eu_x = euler_angles(1);
eu_y = euler_angles(2);
eu_z = euler_angles(3);

R = [cos(eu_y)*cos(eu_z); -cos(eu_y)*sin(eu_z); sin(eu_y); ...
    cos(eu_x)*sin(eu_z)+sin(eu_x)*sin(eu_y)*cos(eu_z); cos(eu_x)*cos(eu_z)-sin(eu_x)*sin(eu_y)*sin(eu_z); -sin(eu_x)*cos(eu_y); ...
    sin(eu_x)*sin(eu_z)-cos(eu_x)*sin(eu_y)*cos(eu_z); sin(eu_x)*cos(eu_z)+cos(eu_x)*sin(eu_y)*sin(eu_z); cos(eu_x)*cos(eu_y)];
% R is 1x9

R_unflattened = UKF.unflatten_matrix(R);
q = rotm2quat(R_unflattened)';
      


end

== matlab function controller_v13/Adaptive Controller/observer/UKF/UKF2/pack measurement vector ==
  data: r input; z_raw output; q input; r_dot input; omega input
function z_raw = fcn(r, q, r_dot, omega)
    z_raw = vertcat(r, q, r_dot, omega);
end

== matlab function controller_v13/Adaptive Controller/observer/UKF/UKF2/quaternion to rotation matrix ==
  data: q input; R_flat output
function R_flat = fcn(q)
    % Assume q = [q_s; q_x, q_y, q_z];
    R = quat2rotm(q');
    R_flat = UKF.flatten_matrix(R);
end

== matlab function controller_v13/Adaptive Controller/observer/UKF/UKF2/unpack state vector ==
  data: s input; r output; q output; r_dot output; omega output
function [r, q, r_dot, omega] = fcn(s)
    [r, q, r_dot, omega] = UKF.partial_unpack_s(s);
end

== matlab function controller_v13/Adaptive Controller/observer/UKF/eul to rotation matrix ==
  data: euler_angles input; R output
function R = fcn(euler_angles)
%#codegen

eu_x = euler_angles(1);
eu_y = euler_angles(2);
eu_z = euler_angles(3);

R = [cos(eu_y)*cos(eu_z); -cos(eu_y)*sin(eu_z); sin(eu_y); ...
    cos(eu_x)*sin(eu_z)+sin(eu_x)*sin(eu_y)*cos(eu_z); cos(eu_x)*cos(eu_z)-sin(eu_x)*sin(eu_y)*sin(eu_z); -sin(eu_x)*cos(eu_y); ...
    sin(eu_x)*sin(eu_z)-cos(eu_x)*sin(eu_y)*cos(eu_z); sin(eu_x)*cos(eu_z)+cos(eu_x)*sin(eu_y)*sin(eu_z); cos(eu_x)*cos(eu_y)];
% R is 1x9 (actually 9x1)
% euler_angles: assuming r, p, y
% euler_angles = euler_angles(:)';
% R = eul2rotm(euler_angles);
end

== matlab function controller_v13/MATLAB Function1 ==
  data: u input; y output
function y = fcn(u)

y = u;

== matlab function controller_v13/Force//Torque to Trajectory Specs/nominal desired voltage/force to voltage (sommersault)/MATLAB Function1 ==
  data: u input; y output; rbt parameter; ctr parameter
function y = fcn(u,rbt,ctr)


% Very import: saturate inputs of polynomial!
% No guarantee of monotonicity! 
u_ub = ones(4,1)*ctr.lim.unit_force.ub;
u_lb = ones(4,1)*ctr.lim.unit_force.lb;

% apply saturation
u = max(min(u(:), u_ub(:)), u_lb(:));

y = polyval(rbt.thrust_to_voltage_polyfit, u);

end

== matlab function controller_v13/Adaptive Controller/observer/Rotm2rpy1 ==
  data: R input; rpy output size=3
function rpy   = fcn(R)
    R = unflatten_rotm(R);
    temp = rotm2eul(R, 'XYZ'); 
    rpy = temp(:);
    %rpy = [ypr(3); ypr(2); ypr(1)];
end

== matlab function controller_v13/Adaptive Controller/Attitude and thrust learned NMPC/Learned RTNMPC ==
  data: B_omega_d output; f_cmd output; r input; r_dot input; r_dotdot input; R input; Omega input; rd input; rd_d input; rd_dd input; rd_ddd input; rd_dddd input; int_e input; q_prev input; r_origin input; time input; ctr parameter; rbt parameter; mdl parameter; x_in output; u output; obs output; ypr_WI output; ypr_IB output; ypr_WB output; q output; r_origin output; time output
function [B_omega_d, f_cmd, x_in, u, obs, ypr_WI, ypr_IB, ypr_WB, q, r_origin, time] = fcn(r, r_dot, r_dotdot, R,  Omega, rd, rd_d, rd_dd, rd_ddd, rd_dddd, int_e, q_prev, r_origin, time, ctr, rbt, mdl)
    %#codegen
    % r: curr pos
    % r_dot: curr vel
    % R: current attitude
    % Omega: current body rates
    % rd : des pos
    % rd_d: des vel
    %% Out: 
    % cmd_B_thrust_z is thrust force on z axis in body (B) frame [N]
    
    % Ensure signals have expected shape
    R = unflatten_rotm(R(:));    % rotation matrix

    % Angular velocity
    Omega = Omega(:);               % ang vel [rad/s]

    % Position and velocity
    r = r(:);                       % position [m]
    r_dot = r_dot(:);               % velocity [m/s]

    % Policy-specific variables (move out)
    %r0_policy = [0.0; 0.0; 0.1];    % this is the origin for the learned policy in [m]
    r0_policy = ctr.rtnmpc.r0_policy;
    f_ext = zeros(3,1);             % TODO : in the future, f_ext will need to be converted in "bee" units

    % Compute yaw-fixed reference frame
    R_IB = eye(3); % needed by simulink compiler
    R_WI = eye(3);
    if ctr.rtnmpc.yaw_fixed_frame.en
        [R_WI, R_IB] = compute_yaw_fixed_frame(R, ctr.rtnmpc.yaw_fixed_framw.align_on_x);
    
        % Compute attitude quaternion
        q = quat_scalar_last_from_rotm(R_WI);

        % logging
        ypr_WI = rotm2eul(R_WI)';
        ypr_IB = rotm2eul(R_IB)';
        ypr_WB = rotm2eul(R)';
    else
        q = quat_scalar_last_from_rotm(R);

        ypr_WI = rotm2eul(eye(3))';
        ypr_IB = rotm2eul(eye(3))';
        ypr_WB = rotm2eul(R)';
    end

    % Kusaka, Takashi, and Takayuki Tanaka. "Stateful Rotor for Continuity 
    % of Quaternion and Fast Sensor Fusion Algorithm Using 9-Axis Sensors." 
    % Sensors 22.20 (2022): 7989.
    q = sign(q'*q_prev)*q; % stateful rotor
    
    if time < 0
        r_origin = r;
    end

    % Set current state
    x = [r(:) + r0_policy(:) - r_origin(:) - ctr.rtmpc.r_origin_offset; r_dot; q;]; % [m, m, m, m/s, m/s, m/s, 1-norm, ..., 1-norm]
    x_in = x(:).*ctr.rtmpc.in_scaling(1:10); % column vector; convert to "bee" units [dm, ..., dm, dm/s, ..., dm/s, 1-norm, ..., 1-norm]
    
    % Call NN policy
    obs = [x_in(:); f_ext; max(time,0)]/ctr.rtmpc.max_obs; % column vector; convert to "bee" units
    
    u_as_float = ctr.rtmpc.max_act*ctr.rtmpc.out_scaling.*rtmpcnn(obs, ctr.rtmpc.nnparam); % ub -1, 1
    u = cast(u_as_float, 'double');

    % Advance to next timestep - until done
    time = min(time + mdl.T, ctr.rtmpc.t_max);

    m = rbt.m;
    g = mdl.g;
    
    u = u(:);
    
    % saturate control inputs for safety
    u_lim = [ctr.rtmpc.lim.omega; ctr.rtmpc.lim.omega; ctr.rtmpc.lim.omega; ctr.rtmpc.lim.f_cmd_norm];
    u = max(min(u, u_lim), -u_lim);
    
    % unpack control inputs
    I_omega_d = u(1:3);         % in [rad/s]
    f_cmd_normalized = u(4);    % in -1, 1
    
    % I_omega_d(2) = 0.0; % TODO: ANDREA: TUNE AND REMOVE THIS

    if ctr.rtnmpc.yaw_fixed_frame.en
        B_omega_d = R_IB'*I_omega_d;
    else
        B_omega_d = I_omega_d;
    end
    B_omega_d(3) = 0.0; % no commands on z :(
    
    % thust force
    f_cmd = m * g * (1.0 + f_cmd_normalized); % in [N]

end

function q = quat_scalar_last_from_rotm(R)

    % Compute attitude quaterniona from rotation matrix
    % and ensure positive scalar part
    q_wxyz = rotm2quat(R);  % scalar first
    q_wxyz = q_wxyz(:);
    q = [q_wxyz(2:4); q_wxyz(1)]; 

end

== matlab function controller_v13/Force//Torque to Trajectory Specs/nominal desired voltage/force to voltage (sommersault)/MATLAB Function ==
  data: Vi input; Vo output; mdl parameter
function Vo = fcn(Vi,mdl)
%old script
% if max(Vi)>mdl.max_v
%     Vo = Vi * mdl.max_v/max(Vi);
%     % scale down all votages if one exceeds the max limit.
% else
%     Vo = Vi;
% end

%new change (modify max_v to a vector so each DEA has its own max)
% scale_down_ratio_vec = Vi ./ mdl.max_v_vec;
% scale_down_ratio = max(scale_down_ratio_vec);
% bool_scale_down = scale_down_ratio>1;
% 
% if bool_scale_down
%    Vo = Vi/scale_down_ratio;
% else
%    Vo = Vi; 
% end

%%%%%%%%%%%%%%%%%%%%%%%%%%%%%%%%%%%%%%%%%%%%%%%%%%%%%%%%%%%%%%%%%%

% min_v_vec = mdl.hovering_vec -150;
% scale_down_ratio_vec = (Vi-min_v_vec)./(mdl.max_v_vec-min_v_vec);
% 
% scale_down_ratio = max(scale_down_ratio_vec);
% bool_scale_down = scale_down_ratio>1;
% 
% if bool_scale_down
%     Vo = min_v_vec + (Vi - min_v_vec)./scale_down_ratio;	
% else
% 	Vo = Vi; 
% end

Vo = Vi; 

%extra layer of safety
for i=1:length(Vo)
	Vo(i) = min(Vo(i),mdl.max_v_vec(i));
end
